simulink model "final_quadruped_200522"  (R2021a)
settings: Solver=ode15s  StartTime=0.0  StopTime=1  RelTol=1e-3  EnableMultiTasking=on
values from neighbouring files (symbols this model uses):
  foot_x = 8    [bipedparameters.m]    (also in fcn.m; finalrobotParameters.m; finalrobotParameters_110522.m; finalrobotParameters_140522.m)
  foot_y = 6    [bipedparameters.m]    (also in fcn.m; finalrobotParameters.m; finalrobotParameters_110522.m; finalrobotParameters_140522.m)
  foot_z = 1    [bipedparameters.m]    (also in fcn.m; finalrobotParameters.m; finalrobotParameters_110522.m; finalrobotParameters_140522.m)
  height_plane = 0.025    [bipedparameters.m]    (also in finalrobotParameters.m; finalrobotParameters_110522.m; finalrobotParameters_140522.m; finalrobotParameters_240522.m)
  kd = 1000    [bipedparameters.m]    (also in finalrobotParameters_140522.m = 5; finalrobotParameters_240522.m)
  ki = 1000    [bipedparameters.m]    (also in finalrobotParameters_140522.m = 5; finalrobotParameters_240522.m)
  kp = 1000    [bipedparameters.m]    (also in finalrobotParameters_140522.m = 5; finalrobotParameters_240522.m)
  lower_leg_length = 10    [bipedparameters.m]    (also in fcn.m; finalrobotParameters.m; finalrobotParameters_110522.m; finalrobotParameters_140522.m)
  m_ll = density*leg_radius*leg_radius*lower_leg_length*3.141592653589*0.01*0.01*0.01    (= 0.0176714586764)    [bipedparameters.m]    (also in fcn.m; finalrobotParameters_140522.m; finalrobotParameters_240522.m; hdotlb.m)
  m_ul = density*leg_radius*leg_radius*upper_leg_length*3.141592653589*0.01*0.01*0.01    (= 0.0176714586764)    [bipedparameters.m]    (also in fcn.m; finalrobotParameters_140522.m; finalrobotParameters_240522.m; hdotlb.m)
  plane_x = 25    [bipedparameters.m]    (also in finalrobotParameters.m; finalrobotParameters_110522.m; finalrobotParameters_140522.m; finalrobotParameters_240522.m)
  plane_y = 3    [bipedparameters.m]    (also in finalrobotParameters.m; finalrobotParameters_110522.m; finalrobotParameters_140522.m; finalrobotParameters_240522.m)
  torso_offset_x = -0.5    [bipedparameters.m]    (also in finalrobotParameters.m = 10; finalrobotParameters_110522.m = 10; finalrobotParameters_140522.m = 10; finalrobotParameters_240522.m = 10)
  torso_offset_z = -2    [bipedparameters.m]    (also in finalrobotParameters.m; finalrobotParameters_110522.m; finalrobotParameters_140522.m; finalrobotParameters_240522.m)
  torso_x = 5    [bipedparameters.m]    (also in fcn.m = 25; finalrobotParameters.m = 25; finalrobotParameters_110522.m = 25; finalrobotParameters_140522.m = 25)
  torso_y = 10    [bipedparameters.m]    (also in fcn.m = 16; finalrobotParameters.m = 16; finalrobotParameters_110522.m = 16; finalrobotParameters_140522.m = 16)
  torso_z = 8    [bipedparameters.m]    (also in fcn.m = 10; finalrobotParameters.m = 10; finalrobotParameters_110522.m = 10; finalrobotParameters_140522.m = 10)
  upper_leg_length = 10    [bipedparameters.m]    (also in fcn.m; finalrobotParameters.m; finalrobotParameters_110522.m; finalrobotParameters_140522.m)
undefined symbols (not defined in the file or in its folder): X, Y, Z
libraries: nesl_utility x102, sm_lib x71, Contact_Forces_Lib x16, pid_lib x12, fl_lib x4
(part 7 of 7)

== matlab function final_quadruped_200522/Model/Left Leg Front/Subsystem/MATLAB Function4 ==
  data: eb1g input; eb2g input; ab1g input; ab2g input; eb3g input; vlinks input; w_torso input; eb_dg1 output; td1 input; v_torso input; eb_dg2 output; td2 input; td3 input; eb_dg3 output; rho_dotLF output
function [eb_dg1,eb_dg2,eb_dg3,rho_dotLF] = fcn(eb1g,eb2g,ab1g,ab2g, eb3g, vlinks, w_torso, td1, v_torso, td2, td3)
w0=w_torso;
w1=w0+eb1g*td1;
w2=w1+eb2g*td2;
w3=w2+eb3g*td3;

eb_dg1=cross(w1,eb1g);
eb_dg2=cross(w2,eb2g);
eb_dg3=cross(w3,eb3g);


vcf=zeros(3,3);
vof=zeros(3,3);
rho_dotLF=zeros(3,3,3);
vcf(:,1)=vlinks(4);
vcf(:,2)=vlinks(5);
vcf(:,3)=vlinks(6);
vof(:,1)=v_torso;
vof(:,2)=vof(:,1)+cross(w1,ab1g);
vof(:,3)=vof(:,2)+cross(w2,ab2g);
for i=1:3
    for j=1:3
        if j<i
rho_dotLF(:,j,i)=zeros(3,1);
        else
rho_dotLF(:,j,i)=vcf(:,j)-vof(:,i);
        end
    end
end

end

== matlab function final_quadruped_200522/Model/Right Leg Back/Subsystem/MATLAB Function2 ==
  data: h_dotRB output; ec_dg1 input; ec1g input; ec2g input; ec3g input; ec_dg2 input; ec_dg3 input; rho_dotRB input; rhoRB input
function h_dotRB = fcn( ec_dg1,ec1g, ec2g, ec3g, ec_dg2, ec_dg3, rho_dotRB, rhoRB)
%%
lower_leg_length = 10;
upper_leg_length = 10;
density = 1000;
foot_density=2000;
leg_radius = 0.75;
foot_x = 8;
foot_y = 6;
foot_z = 1;
m_ul=density*leg_radius*leg_radius*upper_leg_length*3.141592653589*0.01*0.01*0.01;
m_ll=density*leg_radius*leg_radius*lower_leg_length*3.141592653589*0.01*0.01*0.01;
m_foot=foot_density*foot_x*foot_y*foot_z*0.000001;

%%
h1_dot=(m_ul*cross(ec1g,rho_dotRB(:,1,1)))+(m_ul*cross(ec_dg1,rhoRB(:,1,1)))+(m_ll*cross(ec1g,rho_dotRB(:,2,1)))+(m_ll*cross(ec_dg1,rhoRB(:,2,1)))+(m_foot*cross(ec1g,rho_dotRB(:,3,1)))+(m_foot*cross(ec_dg1,rhoRB(:,3,1)));
h2_dot=(m_ll*cross(ec2g,rho_dotRB(:,2,2)))+(m_ll*cross(ec_dg2,rhoRB(:,2,2)))+(m_foot*cross(ec2g,rho_dotRB(:,3,2)))+(m_foot*cross(ec_dg2,rhoRB(:,3,2)));
h3_dot=m_foot*(cross(ec3g,rho_dotRB(:,3,3)))+m_foot*(cross(ec_dg3,rhoRB(:,3,3)));

h_dotRB =[h1_dot h2_dot h3_dot];



end

== matlab function final_quadruped_200522/Model/Right Leg Back/Subsystem/MATLAB Function4 ==
  data: ec1g input; ec2g input; ac1g input; ac2g input; ec3g input; vlinks input; w_torso input; ec_dg1 output; td1 input; v_torso input; ec_dg2 output; td2 input; td3 input; ec_dg3 output; rho_dotRB output
function [ec_dg1,ec_dg2,ec_dg3,rho_dotRB] = fcn(ec1g,ec2g,ac1g,ac2g, ec3g, vlinks, w_torso, td1, v_torso, td2, td3)
w0=w_torso;
w1=w0+ec1g*td1;
w2=w1+ec2g*td2;
w3=w2+ec3g*td3;

ec_dg1=cross(w1,ec1g);
ec_dg2=cross(w2,ec2g);
ec_dg3=cross(w3,ec3g);


vcf=zeros(3,3);
vof=zeros(3,3);
rho_dotRB=zeros(3,3,3);
vcf(:,1)=vlinks(4);
vcf(:,2)=vlinks(5);
vcf(:,3)=vlinks(6);
vof(:,1)=v_torso;
vof(:,2)=vof(:,1)+cross(w1,ac1g);
vof(:,3)=vof(:,2)+cross(w2,ac2g);
for i=1:3
    for j=1:3
        if j<i
rho_dotRB(:,j,i)=zeros(3,1);
        else
rho_dotRB(:,j,i)=vcf(:,j)-vof(:,i);
        end
    end
end

end

== matlab function final_quadruped_200522/Model/Left LegBack/Subsystem/MATLAB Function2 ==
  data: h_dotLB output; ed_dg1 input; ed1g input; ed2g input; ed3g input; ed_dg2 input; ed_dg3 input; rho_dotLB input; rhoLB input
function h_dotLB = fcn( ed_dg1,ed1g, ed2g, ed3g, ed_dg2, ed_dg3, rho_dotLB, rhoLB)
%%
lower_leg_length = 10;
upper_leg_length = 10;
density = 1000;
foot_density=2000;
leg_radius = 0.75;
foot_x = 8;
foot_y = 6;
foot_z = 1;
m_ul=density*leg_radius*leg_radius*upper_leg_length*3.141592653589*0.01*0.01*0.01;
m_ll=density*leg_radius*leg_radius*lower_leg_length*3.141592653589*0.01*0.01*0.01;
m_foot=foot_density*foot_x*foot_y*foot_z*0.000001;

%%
h1_dot=(m_ul*cross(ed1g,rho_dotLB(:,1,1)))+(m_ul*cross(ed_dg1,rhoLB(:,1,1)))+(m_ll*cross(ed1g,rho_dotLB(:,2,1)))+(m_ll*cross(ed_dg1,rhoLB(:,2,1)))+(m_foot*cross(ed1g,rho_dotLB(:,3,1)))+(m_foot*cross(ed_dg1,rhoLB(:,3,1)));
h2_dot=(m_ll*cross(ed2g,rho_dotLB(:,2,2)))+(m_ll*cross(ed_dg2,rhoLB(:,2,2)))+(m_foot*cross(ed2g,rho_dotLB(:,3,2)))+(m_foot*cross(ed_dg2,rhoLB(:,3,2)));
h3_dot=m_foot*(cross(ed3g,rho_dotLB(:,3,3)))+m_foot*(cross(ed_dg3,rhoLB(:,3,3)));

h_dotLB =[h1_dot h2_dot h3_dot];



end

== matlab function final_quadruped_200522/Subsystem/MATLAB Function2 ==
  data: vx input; vy input; v output; vz input
function v = fcn(vx,vy,vz)
v=[vx;vy;vz];
end

== matlab function final_quadruped_200522/Model/Left LegBack/Subsystem/MATLAB Function4 ==
  data: ed1g input; ed2g input; ad1g input; ad2g input; ed3g input; vlinks input; w_torso input; ed_dg1 output; td1 input; v_torso input; ed_dg2 output; td2 input; td3 input; ed_dg3 output; rho_dotLB output
function [ed_dg1,ed_dg2,ed_dg3,rho_dotLB] = fcn(ed1g,ed2g,ad1g,ad2g, ed3g, vlinks, w_torso, td1, v_torso, td2, td3)
w0=w_torso;
w1=w0+ed1g*td1;
w2=w1+ed2g*td2;
w3=w2+ed3g*td3;

ed_dg1=cross(w1,ed1g);
ed_dg2=cross(w2,ed2g);
ed_dg3=cross(w3,ed3g);


vcf=zeros(3,3);
vof=zeros(3,3);
rho_dotLB=zeros(3,3,3);
vcf(:,1)=vlinks(4);
vcf(:,2)=vlinks(5);
vcf(:,3)=vlinks(6);
vof(:,1)=v_torso;
vof(:,2)=vof(:,1)+cross(w1,ad1g);
vof(:,3)=vof(:,2)+cross(w2,ad2g);
for i=1:3
    for j=1:3
        if j<i
rho_dotLB(:,j,i)=zeros(3,1);
        else
rho_dotLB(:,j,i)=vcf(:,j)-vof(:,i);
        end
    end
end

end

== matlab function final_quadruped_200522/Model/Left Leg Front/MATLAB Function1 ==
  data: ankle input; knee input; t2dRF output; hip input
function t2dRF= fcn(ankle, knee, hip)
t2dRF=[hip;knee;ankle];
end

== matlab function final_quadruped_200522/Model/Right Leg Front /MATLAB Function1 ==
  data: ankle input; knee input; t2dRF output; hip input
function t2dRF= fcn(ankle, knee, hip)
t2dRF=[hip;knee;ankle];
end

== matlab function final_quadruped_200522/MATLAB Function2 ==
  data: ax input; a_torso output; ay input; az input
function a_torso = fcn(ax, ay, az)
a_torso=[ax; ay; az];
end

== matlab function final_quadruped_200522/Model/Left Leg Front/Contact Forces /MATLAB Function ==
  data: n1 input; NLF output; n2 input; n4 input; n3 input; f1 input; f2 input; f3 input; f4 input; FLF output
function [NLF,FLF] = fcn(n1,n2,n4,n3,f1,f2,f3,f4)
% mu_s = 0.8;
% alpha=atan(mu_s);
% NRF=n1+n2+n3+n4;
% FRFca=f1*cos(alpha)+f2*cos(alpha)+f3*cos(alpha)+f4*cos(alpha);
% FRFsa=f1*sin(alpha)+f2*sin(alpha)+f3*sin(alpha)+f4*sin(alpha);
NLF=n1+n2+n3+n4;
FLF=f1+f2+f3+f4;
end

== matlab function final_quadruped_200522/Model/MATLAB Function2 ==
  data: theta_d_des input; theta_2d_des output; h_dot input; h input; a_torso input; M input; f input
function theta_2d_des = fcn(theta_d_des, h_dot, h, a_torso, M, f)
g=[0; 0; -9.80665];
theta_2d_des=-pinv(h)*((-h_dot*theta_d_des)-M*a_torso+M*g-f);
-h_dot*theta_d_des
end

== matlab function final_quadruped_200522/Model/Right Leg Front /Contact Forces /MATLAB Function ==
  data: n1 input; NRF output; n2 input; n4 input; n3 input; f1 input; f2 input; f3 input; f4 input; FRF output
function [NRF,FRF] = fcn(n1,n2,n4,n3,f1,f2,f3,f4)
% mu_s = 0.8;
% alpha=atan(mu_s);
% NRF=n1+n2+n3+n4;
% FRFca=f1*cos(alpha)+f2*cos(alpha)+f3*cos(alpha)+f4*cos(alpha);
% FRFsa=f1*sin(alpha)+f2*sin(alpha)+f3*sin(alpha)+f4*sin(alpha);
NRF=n1+n2+n3+n4;
FRF=f1+f2+f3+f4;
end

== matlab function final_quadruped_200522/Subsystem/MATLAB Function3 ==
  data: vx input; vy input; v output; vz input
function v = fcn(vx,vy,vz)
v=[vx;vy;vz];
end

== matlab function final_quadruped_200522/Model/Right Leg Back/Contact Forces /MATLAB Function ==
  data: n1 input; NRB output; n2 input; n4 input; n3 input; f1 input; f2 input; f3 input; f4 input; FRB output
function [NRB,FRB] = fcn(n1,n2,n4,n3,f1,f2,f3,f4)
% mu_s = 0.8;
% alpha=atan(mu_s);
% NRF=n1+n2+n3+n4;
% FRFca=f1*cos(alpha)+f2*cos(alpha)+f3*cos(alpha)+f4*cos(alpha);
% FRFsa=f1*sin(alpha)+f2*sin(alpha)+f3*sin(alpha)+f4*sin(alpha);
NRB=n1+n2+n3+n4;
FRB=f1+f2+f3+f4;
end

== matlab function final_quadruped_200522/Model/Left LegBack/Contact Forces /MATLAB Function ==
  data: n1 input; NLB output; n2 input; n4 input; n3 input; f1 input; f2 input; f3 input; f4 input; FLB output
function [NLB,FLB] = fcn(n1,n2,n4,n3,f1,f2,f3,f4)
% mu_s = 0.8;
% alpha=atan(mu_s);
% NRF=n1+n2+n3+n4;
% FRFca=f1*cos(alpha)+f2*cos(alpha)+f3*cos(alpha)+f4*cos(alpha);
% FRFsa=f1*sin(alpha)+f2*sin(alpha)+f3*sin(alpha)+f4*sin(alpha);
NLB=n1+n2+n3+n4;
FLB=f1+f2+f3+f4;
end

== matlab function final_quadruped_200522/Model/MATLAB Function3 ==
  data: NRF input; f output; FRF input; NLF input; FLF input; NRB input; FRB input; NLB input; FLB input
function f = fcn(NRF,FRF,NLF,FLF,NRB,FRB, NLB,FLB)
N=NRF+NLF+NRB+NLB;
F=FRF+FLF+FRB+FLB;
f=[F(1);F(2); N+F(3)];
end

== matlab function final_quadruped_200522/Model/Right Leg Front /Subsystem/MATLAB Function ==
  data: ea1g output; ea2g output; ea3g output; qha input; qaa input; Qquat input; qka input; aa1g output; aa2g output; cma1g output; cma2g output; cma3g output
function [ea1g,ea2g,ea3g,aa1g,aa2g,cma1g,cma2g,cma3g] = fcn(qha,qaa,Qquat,qka)
%%
lower_leg_length = 10;
upper_leg_length = 10;
foot_offset=[-1; 0; 0];

%%
disp(Qquat);
Qquat
Qd0g=quat2rotm([Qquat(1) Qquat(2) Qquat(3) Qquat(4)]);
Qd10=[cos(qha) 0 sin(qha);
      0 1 0 ;
      -sin(qha) 0 cos(qha)];
Qd1g=Qd10*Qd0g;
  
Qd21=[cos(qka) 0 sin(qka);
      0 1 0 ;
      -sin(qka) 0 cos(qka)];
  
Qd32=[1 0 0;
      0 cos(qaa) -sin(qaa);
      0 sin(qaa) cos(qaa)];
  
Qd20 = Qd21* Qd10;
Qd30=Qd32*Qd20;
Qd2g=Qd20*Qd0g;
Qd3g=Qd30*Qd0g;

%axis in local frames
ed1l=[0;
      1;
      0];
ed2l=[0;
      1;
      0];
ed3l=[0;
     0;
     1];
  
%link vector in local frame
ad1l=[0;
      0;
      -upper_leg_length];
   
ad2l=[0;
      0;
      -lower_leg_length];
         
%axis in global frames
ea1g = Qd1g*ed1l;
ea2g = Qd2g*ed2l;
ea3g = Qd3g*ed3l;

%link vector in global frame
aa1g = Qd1g*ad1l;
aa2g = Qd2g*ad2l;

%COM distances in base frame
cma1g=aa1g/2;
cma2g=aa2g/2;
cma3g=Qd3g*foot_offset;


end

== matlab function final_quadruped_200522/Model/Left Leg Front/Subsystem/MATLAB Function ==
  data: eb1g output; eb2g output; eb3g output; qhb input; qab input; Qquat input; qkb input; ab1g output; ab2g output; cmb1g output; cmb2g output; cmb3g output
function [eb1g,eb2g,eb3g,ab1g,ab2g,cmb1g,cmb2g,cmb3g] = fcn(qhb,qab,Qquat,qkb)
%%
lower_leg_length = 10;
upper_leg_length = 10;
foot_offset=[-1; 0; 0];

%%
Qd10=zeros(3,3);
% disp(Qquat);
% Qquat=reshape(Qquat,4,1);
Qquat;
Qd0g=quat2rotm([Qquat(1) Qquat(2) Qquat(3) Qquat(4)]);
% Qd0geul=quat2eul(Qquat);
% Qd0g=eul2rotm(Qd0geul);
Qd10=[cos(qhb) 0 sin(qhb);
      0 1 0 ;
      -sin(qhb) 0 cos(qhb)];
Qd1g=Qd10*Qd0g;
  
Qd21=[cos(qkb) 0 sin(qkb);
      0 1 0 ;
      -sin(qkb) 0 cos(qkb)];
  
Qd32=[1 0 0;
      0 cos(qab) -sin(qab);
      0 sin(qab) cos(qab)];
  
Qd20 = Qd21* Qd10;
Qd30=Qd32*Qd20;
Qd2g=Qd20*Qd0g;
Qd3g=Qd30*Qd0g;

%axis in local frames
ed1l=[0;
      1;
      0];
ed2l=[0;
      1;
      0];
ed3l=[0;
     0;
     1];
  
%link vector in local frame
ad1l=[0;
      0;
      -upper_leg_length];
   
ad2l=[0;
      0;
      -lower_leg_length];
         
%axis in global frames
eb1g = Qd1g*ed1l;
eb2g = Qd2g*ed2l;
eb3g = Qd3g*ed3l;

%link vector in global frame
ab1g = Qd1g*ad1l;
ab2g = Qd2g*ad2l;

%COM distances in base frame
cmb1g=ab1g/2;
cmb2g=ab2g/2;
cmb3g=Qd3g*foot_offset;


end
